simulink model "OEW_PMSM_DI_SVPWM_ZSC_Control"  (R2022b)
settings: Solver=FixedStepAuto  StartTime=0.0  StopTime=0.3  FixedStep=Ts  RelTol=1e-3
model workspace (MAT data in the model file):
  B = Simulink.Parameter
  B.Value = 0.002
  B.DataType = 'auto'
  B.Complexity = 'real'
  B.Dimensions = [1 1]
  J = Simulink.Parameter
  J.Value = 0.001
  J.DataType = 'auto'
  J.Complexity = 'real'
  J.Dimensions = [1 1]
  L0 = Simulink.Parameter
  L0.Value = 0.001
  L0.DataType = 'auto'
  L0.Complexity = 'real'
  L0.Dimensions = [1 1]
  Ld = Simulink.Parameter
  Ld.Value = 0.00176
  Ld.DataType = 'auto'
  Ld.Complexity = 'real'
  Ld.Dimensions = [1 1]
  Lq = Simulink.Parameter
  Lq.Value = 0.00176
  Lq.DataType = 'auto'
  Lq.Complexity = 'real'
  Lq.Dimensions = [1 1]
  Rs = Simulink.Parameter
  Rs.Value = 0.2
  Rs.DataType = 'auto'
  Rs.Complexity = 'real'
  Rs.Dimensions = [1 1]
  flux = Simulink.Parameter
  flux.Value = 0.1688
  flux.DataType = 'auto'
  flux.Complexity = 'real'
  flux.Dimensions = [1 1]
  flux_3 = Simulink.Parameter
  flux_3.Value = 0.006
  flux_3.DataType = 'auto'
  flux_3.Complexity = 'real'
  flux_3.Dimensions = [1 1]
  pn = Simulink.Parameter
  pn.Value = 4
  pn.DataType = 'auto'
  pn.Complexity = 'real'
  pn.Dimensions = [1 1]
undefined symbols (not defined in the file): DiscIntNeverNeededParam, Tpwm, Ts, Tsample, Tspeed, Udc
libraries: spsControlledCurrentSourceLib x3, spsVoltageMeasurementLib x3, slpidlib x3, spsUniversalBridgeLib x2, spsDCVoltageSourceLib x1, simulink x1, spsSecondOrderFilterLib x1, sps_lib x1
settings Model: DataDictionary=OEW_PMSM_DI_SVPWM_ZSC_Control.sldd  Creator=SSC  LastModifiedBy=SSC

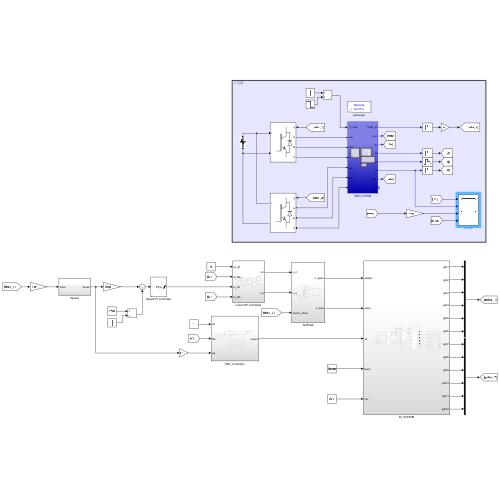
[thumbnail: Simulink's stored preview of the top-level diagram]
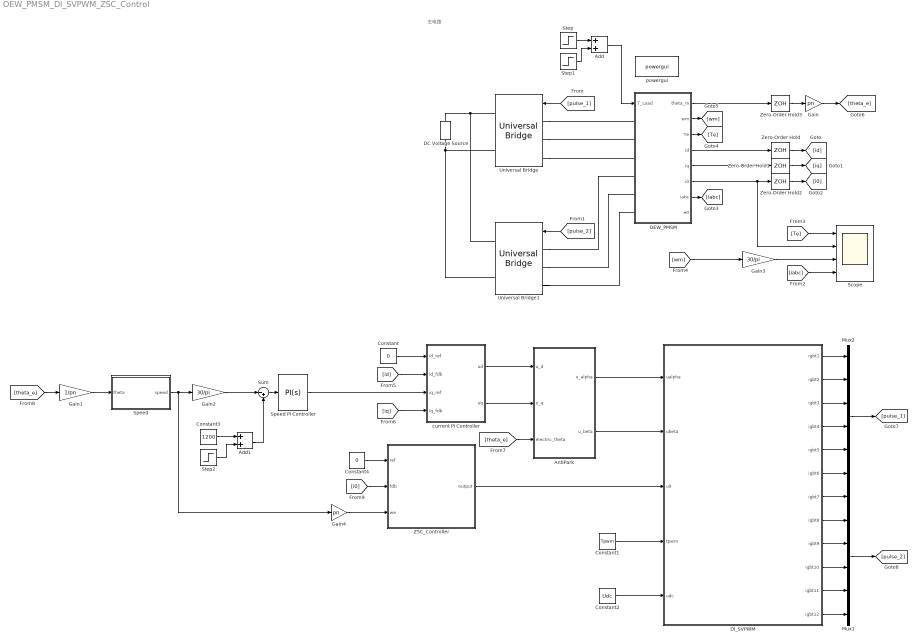
== system OEW_PMSM_DI_SVPWM_ZSC_Control ==
  note: 主电路
  Add : Sum
  Add1 : Sum
  AntiPark : Subsystem
  Constant : Constant  Value=0
  Constant1 : Constant  Value=Tpwm
  Constant2 : Constant  Value=Udc
  Constant3 : Constant  Value=1200
  Constant4 : Constant  Value=0
  DC Voltage Source : spsDCVoltageSourceLib/DC Voltage Source  Amplitude=Udc  Measurements=None
  DI_SVPWM : Subsystem
  Gain : Gain  Gain=pn
  Gain1 : Gain  Gain=1/pn
  Gain2 : Gain  Gain=30/pi
  Gain3 : Gain  Gain=30/pi
  Gain4 : Gain  Gain=pn
  Mux1 : Mux  Inputs=6
  Mux2 : Mux  Inputs=6
  OEW_PMSM : Subsystem
  Scope : Scope  NumInputPorts=4
  Speed : Subsystem
  Speed PI Controller : slpidlib/PID Controller  Controller=PI  Form=Parallel  TimeDomain=Continuous-time  UseExternalTs=off  SampleTime=1e-4  IntegratorMethod=Forward Euler  FilterMethod=Forward Euler  ControllerParametersSource=internal  P=0.1  I=40  UseKiTs=off  D=0  N=100  UseFilter=on  TunerSelectOption=Transfer Function Based (PID Tuner App)  InitialConditionSource=internal  InitialConditionForIntegrator=0  InitialConditionForFilter=0  DifferentiatorICPrevScaledInput=0  ExternalReset=none  TrackingMode=off  Kt=1  LimitOutput=on  SatLimitsSource=internal  UpperSaturationLimit=14  LowerSaturationLimit=-14  LinearizeAsGain=on  AntiWindupMode=clamping  Kb=1  LimitIntegrator=off  UpperIntegratorSaturationLimit=inf  LowerIntegratorSaturationLimit=-inf  POutMin=[]  POutMax=[]  IOutMin=[]  IOutMax=[]  DOutMin=[]  DOutMax=[]  NOutMin=[]  NOutMax=[]  SumOutMin=[]  SumOutMax=[]  SaturationOutMin=[]  SaturationOutMax=[]  PParamMin=[]  PParamMax=[]  IParamMin=[]  IParamMax=[]  DParamMin=[]  DParamMax=[]  NParamMin=[]  NParamMax=[]  KbParamMin=[]  KbParamMax=[]  KtParamMin=[]  KtParamMax=[]  KbOutMin=[]  KbOutMax=[]  KtOutMin=[]  KtOutMax=[]  IntegratorOutMin=[]  IntegratorOutMax=[]  FilterOutMin=[]  FilterOutMax=[]  SumI1OutMin=[]  SumI1OutMax=[]  SumI2OutMin=[]  SumI2OutMax=[]  SumI3OutMin=[]  SumI3OutMax=[]  SumI4OutMin=[]  SumI4OutMax=[]  SumDOutMin=[]  SumDOutMax=[]  DifferentiatorOutMin=[]  DifferentiatorOutMax=[]  FilterDiffOutCoefMin=[]  FilterDiffOutCoefMax=[]  ReciprocalOutMin=[]  ReciprocalOutMax=[]  SumDenOutMin=[]  SumDenOutMax=[]  SumNumOutMin=[]  SumNumOutMax=[]  DivideOutMin=[]  DivideOutMax=[]  UdiffTsProdOutMin=[]  UdiffTsProdOutMax=[]  NTsProdOutMin=[]  NTsProdOutMax=[]  UintegralTsProdOutMin=[]  UintegralTsProdOutMax=[]  UngainTsProdOutMin=[]  UngainTsProdOutMax=[]  ClampingZeroOutDataTypeStr=Inherit: Inherit via back propagation  ClampingZeroOutMin=[]  ClampingZeroOutMax=[]  FilterDenConstantOutDataTypeStr=Inherit: Inherit via back propagation  FilterDenConstantOutMin=[]  FilterDenConstantOutMax=[]  PCopyOutDataTypeStr=Inherit: Inherit via back propagation  PCopyOutMin=[]  PCopyOutMax=[]  NCopyOutDataTypeStr=Inherit: Inherit via back propagation  NCopyOutMin=[]  NCopyOutMax=[]  IntegratorContinuousStateAttributes=''  IntegratorStateMustResolveToSignalObject=off  IntegratorRTWStateStorageClass=Auto  FilterContinuousStateAttributes=''  FilterStateMustResolveToSignalObject=off  FilterRTWStateStorageClass=Auto  ParallelPVariant=InternalParameters  IdealPVariant=Disabled  IVariant=InternalParameters  DVariant=Disabled  IntegratorVariant=Continuous  SatVariant=Enabled  AWVariant=ContClampingParallel  PCopyVariant=Disabled  TRVariant=Disabled  FdbkBlocksVariant=Forward  IdealPFdbkVariant=Disabled  SatFdbkVariant=Disabled  DerivativeFilterVariant=Disabled  NVariant=Disabled  NCopyVariant=Disabled_SignalSpec  FilterICVariant=Disabled  IntegratorICVariant=InternalICs  ExternalResetVariant=Disabled  TRSumVariant=Passthrough  SumFdbkVariant=Disabled  SumVariant=Sum_PI  TsampFilterVariant=InternalTs  TsampNgainVariant=Passthrough  TsampIntegralVariant=Passthrough  ExternalSaturationOutDataTypeStr=Inherit: Same as second input
  Step : Step  Time=0.05  After=12  SampleTime=0
  Step1 : Step  Time=0.12  After=-6  SampleTime=0
  Step2 : Step  Time=0.15  After=-600  SampleTime=0
  Sum : Sum  Inputs=|-+
  Universal Bridge : spsUniversalBridgeLib/Universal Bridge  Arms=3  SnubberResistance=1e5  SnubberCapacitance=inf  Device=IGBT / Diodes  Ron=1e-3  Lon=0  ForwardVoltages="[  0  0  ]"  ForwardVoltage=0  GTOparameters=[ 10e-6 , 20e-6 ]  IGBTparameters=[ 1e-6 , 2e-6 ]  Measurements=None  Measurements_2=None  converterType=Rectifier
  Universal Bridge1 : spsUniversalBridgeLib/Universal Bridge  Arms=3  SnubberResistance=1e5  SnubberCapacitance=inf  Device=IGBT / Diodes  Ron=1e-3  Lon=0  ForwardVoltages="[  0  0  ]"  ForwardVoltage=0  GTOparameters=[ 10e-6 , 20e-6 ]  IGBTparameters=[ 1e-6 , 2e-6 ]  Measurements=None  Measurements_2=None  converterType=Rectifier
  ZSC_Controller : Subsystem
  Zero-Order Hold{,1..3} (4 alike) : ZeroOrderHold  SampleTime=Tsample
  current PI Controller : Subsystem
  powergui : sps_lib/powergui  Priority=1  SimulationMode=Discrete  SampleTime=Ts  frequency=60  Iterations=50  frequencyindice=0  Pbase=100e6  ErrMax=1e-4  UnitsV=kV  UnitsW=MW  buscounter=0  FunctionMessages=off  echomessages=off  EnableUseOfTLC=off  CurrentSourceSwitches=off  DisableSnubberDevices=off  DisableRonSwitches=off  DisableVfSwitches=off  DisplayEquations=off  AutomaticDiscreteSolvers=off  SolverType=Tustin/Backward Euler (TBE)  Interpol=off  ExternalGateDelay=off  methode=off  Ts=100  x0status=blocks  SPID=on  SwTol=0  HookPort=off  NonlinearTolerance=1e-4  nMaxIteration=100  ContinueOnMaxIteration=off  RestoreLinks=warning  ResistiveCurrentMeasurement=off  Frange=[0:2:500]  Ylog=off  Xlog=on  ShowGrid=off  save=off  variable=ZData  structure=0  ZoomFFT=off  StartTime=0.0  cycles=1  DisplayStyle=1  fundamental=60  FreqAxis=off  MaxFrequency=1000  frequencyindicesteady=1  RmsSteady=1  display=off
  wires:
  [pulse_1] -> Universal Bridge/1
  [pulse_2] -> Universal Bridge1/1
  OEW_PMSM/4(id) -> Zero-Order Hold/1
  OEW_PMSM/5(iq) -> Zero-Order Hold1/1
  OEW_PMSM/6(i0) -> Scope/2, Zero-Order Hold2/1
  Zero-Order Hold/1 -> [id]
  Zero-Order Hold1/1 -> [iq]
  Zero-Order Hold2/1 -> [i0]
  OEW_PMSM/7(iabc) -> [iabc]
  [iabc] -> Scope/4
  OEW_PMSM/3(Te) -> [Te]
  [Te] -> Scope/1
  OEW_PMSM/2(wm) -> [wm]
  [wm] -> Gain3/1
  OEW_PMSM/1(theta_m) -> Zero-Order Hold3/1
  Zero-Order Hold3/1 -> Gain/1
  Gain/1 -> [theta_e]
  Step1/1 -> Add/2
  Step/1 -> Add/1
  Add/1 -> OEW_PMSM/1(T_Load)
  Constant/1 -> current PI Controller/1(id_ref)
  [id] -> current PI Controller/2(id_fdb)
  [iq] -> current PI Controller/4(iq_fdb)
  current PI Controller/1(ud) -> AntiPark/1(u_d)
  current PI Controller/2(uq) -> AntiPark/2(u_q)
  [theta_e] -> AntiPark/3(electric_theta)
  AntiPark/1(u_alpha) -> DI_SVPWM/1(ualpha)
  AntiPark/2(u_beta) -> DI_SVPWM/2(ubeta)
  Gain1/1 -> Speed/1(theta)
  [theta_e] -> Gain1/1
  Speed/1(speed) -> Gain4/1, Gain2/1
  Gain2/1 -> Sum/1
  Constant3/1 -> Add1/1
  Sum/1 -> Speed PI Controller/1
  Add1/1 -> Sum/2
  Step2/1 -> Add1/2
  Speed PI Controller/1 -> current PI Controller/3(iq_ref)
  Gain3/1 -> Scope/3
  Constant1/1 -> DI_SVPWM/4(tpwm)
  Constant2/1 -> DI_SVPWM/5(udc)
  DI_SVPWM/12(igbt12) -> Mux1/6
  DI_SVPWM/11(igbt11) -> Mux1/5
  DI_SVPWM/10(igbt10) -> Mux1/4
  DI_SVPWM/9(igbt9) -> Mux1/3
  DI_SVPWM/8(igbt8) -> Mux1/2
  DI_SVPWM/7(igbt7) -> Mux1/1
  DI_SVPWM/6(igbt6) -> Mux2/6
  DI_SVPWM/5(igbt5) -> Mux2/5
  DI_SVPWM/4(igbt4) -> Mux2/4
  DI_SVPWM/3(igbt3) -> Mux2/3
  DI_SVPWM/2(igbt2) -> Mux2/2
  DI_SVPWM/1(igbt1) -> Mux2/1
  Mux2/1 -> [pulse_1]
  Mux1/1 -> [pulse_2]
  ZSC_Controller/1(output) -> DI_SVPWM/3(u0)
  Constant4/1 -> ZSC_Controller/1(ref)
  [i0] -> ZSC_Controller/2(fdb)
  Gain4/1 -> ZSC_Controller/3(we)
  connections:
  Universal Bridge/LConn1 -- OEW_PMSM/LConn1
  Universal Bridge/LConn2 -- OEW_PMSM/LConn2
  Universal Bridge/LConn3 -- OEW_PMSM/LConn3
  Universal Bridge1/LConn1 -- OEW_PMSM/LConn4
  Universal Bridge1/LConn2 -- OEW_PMSM/LConn5
  Universal Bridge1/LConn3 -- OEW_PMSM/LConn6
  DC Voltage Source/LConn1 -- Universal Bridge/RConn2 -- Universal Bridge1/RConn2
  Universal Bridge1/RConn1 -- Universal Bridge/RConn1 -- DC Voltage Source/RConn1

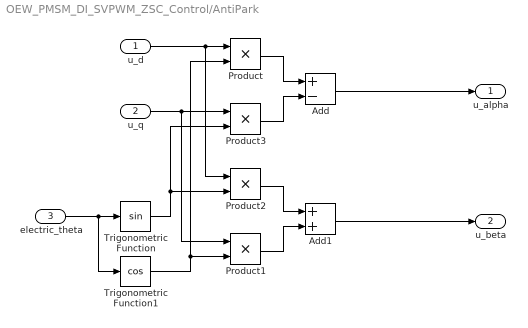
== system OEW_PMSM_DI_SVPWM_ZSC_Control/AntiPark ==
  u_d : Inport
  u_q : Inport  Port=2
  electric_theta : Inport  Port=3
  Add : Sum  Inputs=+-
  Add1 : Sum
  Product{,1..3} (4 alike) : Product
  Trigonometric Function : Trigonometry
  Trigonometric Function1 : Trigonometry  Operator=cos
  u_alpha : Outport
  u_beta : Outport  Port=2
  wires:
  electric_theta/1 -> Trigonometric Function1/1, Trigonometric Function/1
  u_d/1 -> Product2/1, Product/1
  Trigonometric Function1/1 -> Product/2, Product1/2
  u_q/1 -> Product1/1, Product3/1
  Trigonometric Function/1 -> Product2/2, Product3/2
  Product/1 -> Add/1
  Product3/1 -> Add/2
  Add/1 -> u_alpha/1
  Product2/1 -> Add1/1
  Product1/1 -> Add1/2
  Add1/1 -> u_beta/1

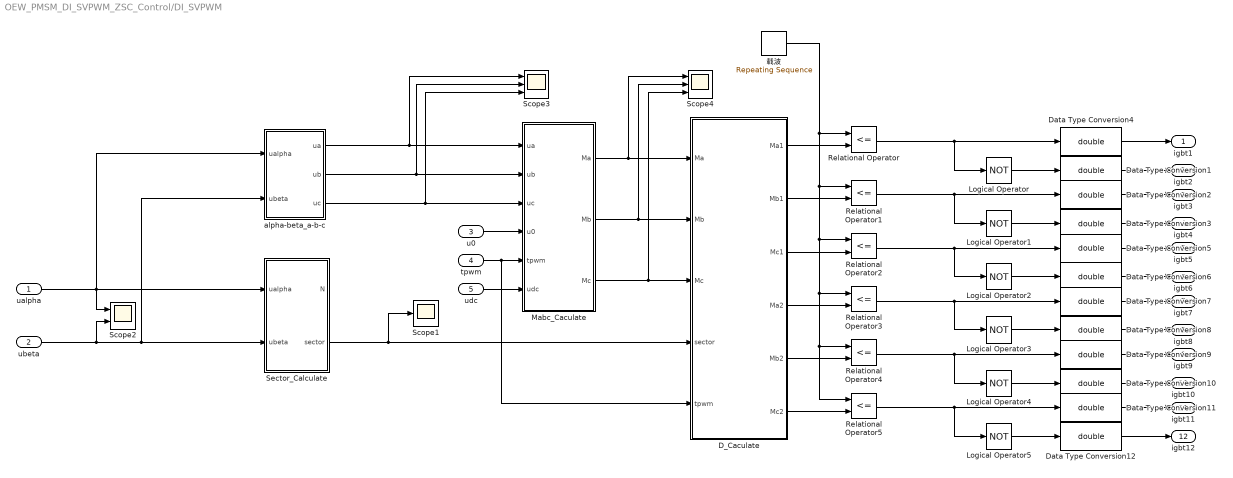
== system OEW_PMSM_DI_SVPWM_ZSC_Control/DI_SVPWM ==
  ualpha : Inport
  ubeta : Inport  Port=2
  u0 : Inport  Port=3
  tpwm : Inport  Port=4
  udc : Inport  Port=5
  D_Caculate : MATLAB Function  TreatAsAtomicUnit=on
  Data Type Conversion{1..12} (12 alike) : DataTypeConversion  OutDataTypeStr=double  SaturateOnIntegerOverflow=off  RndMeth=Floor
  Logical Operator{,1..5} (6 alike) : Logic  Operator=NOT  AllPortsSameDT=off  OutDataTypeStr=boolean
  Mabc_Caculate : MATLAB Function  TreatAsAtomicUnit=on
  Relational Operator{,1..5} (6 alike) : RelationalOperator  Operator=<=  OutDataTypeStr=boolean  RndMeth=Simplest  InputSameDT=off
  Scope1 : Scope
  Scope2 : Scope  NumInputPorts=2
  Scope3 : Scope  NumInputPorts=3
  Scope4 : Scope  NumInputPorts=3
  Sector_Calculate : Subsystem
  alpha-beta_a-b-c : Subsystem
  载波 : simulink/Sources/Repeating Sequence  rep_seq_t=[0 0.5*(1e-4) 1e-4]  rep_seq_y=[0 1e-4 0]
  igbt1 : Outport
  igbt2 : Outport  Port=2
  igbt3 : Outport  Port=3
  igbt4 : Outport  Port=4
  igbt5 : Outport  Port=5
  igbt6 : Outport  Port=6
  igbt7 : Outport  Port=7
  igbt8 : Outport  Port=8
  igbt9 : Outport  Port=9
  igbt10 : Outport  Port=10
  igbt11 : Outport  Port=11
  igbt12 : Outport  Port=12
  wires:
  ubeta/1 -> Scope2/2, alpha-beta_a-b-c/2(ubeta), Sector_Calculate/2(ubeta)
  ualpha/1 -> Scope2/1, Sector_Calculate/1(ualpha), alpha-beta_a-b-c/1(ualpha)
  alpha-beta_a-b-c/1(ua) -> Scope3/1, Mabc_Caculate/1(ua)
  alpha-beta_a-b-c/2(ub) -> Scope3/2, Mabc_Caculate/2(ub)
  alpha-beta_a-b-c/3(uc) -> Scope3/3, Mabc_Caculate/3(uc)
  tpwm/1 -> D_Caculate/5(tpwm), Mabc_Caculate/5(tpwm)
  udc/1 -> Mabc_Caculate/6(udc)
  Mabc_Caculate/1(Ma) -> Scope4/1, D_Caculate/1(Ma)
  Mabc_Caculate/2(Mb) -> Scope4/2, D_Caculate/2(Mb)
  Mabc_Caculate/3(Mc) -> Scope4/3, D_Caculate/3(Mc)
  Sector_Calculate/2(sector) -> D_Caculate/4(sector), Scope1/1
  D_Caculate/1(Ma1) -> Relational Operator/2
  D_Caculate/3(Mc1) -> Relational Operator2/2
  D_Caculate/2(Mb1) -> Relational Operator1/2
  D_Caculate/4(Ma2) -> Relational Operator3/2
  D_Caculate/5(Mb2) -> Relational Operator4/2
  D_Caculate/6(Mc2) -> Relational Operator5/2
  载波/1 -> Relational Operator1/1, Relational Operator2/1, Relational Operator3/1, Relational Operator5/1, Relational Operator4/1, Relational Operator/1
  Relational Operator/1 -> Logical Operator/1, Data Type Conversion4/1
  Logical Operator/1 -> Data Type Conversion1/1
  Relational Operator1/1 -> Logical Operator1/1, Data Type Conversion2/1
  Logical Operator1/1 -> Data Type Conversion3/1
  Relational Operator2/1 -> Logical Operator2/1, Data Type Conversion5/1
  Logical Operator2/1 -> Data Type Conversion6/1
  Relational Operator3/1 -> Logical Operator3/1, Data Type Conversion7/1
  Logical Operator3/1 -> Data Type Conversion8/1
  Relational Operator4/1 -> Logical Operator4/1, Data Type Conversion9/1
  Logical Operator4/1 -> Data Type Conversion10/1
  Relational Operator5/1 -> Logical Operator5/1, Data Type Conversion11/1
  Logical Operator5/1 -> Data Type Conversion12/1
  u0/1 -> Mabc_Caculate/4(u0)
  Data Type Conversion4/1 -> igbt1/1
  Data Type Conversion1/1 -> igbt2/1
  Data Type Conversion2/1 -> igbt3/1
  Data Type Conversion3/1 -> igbt4/1
  Data Type Conversion5/1 -> igbt5/1
  Data Type Conversion6/1 -> igbt6/1
  Data Type Conversion7/1 -> igbt7/1
  Data Type Conversion8/1 -> igbt8/1
  Data Type Conversion9/1 -> igbt9/1
  Data Type Conversion10/1 -> igbt10/1
  Data Type Conversion11/1 -> igbt11/1
  Data Type Conversion12/1 -> igbt12/1

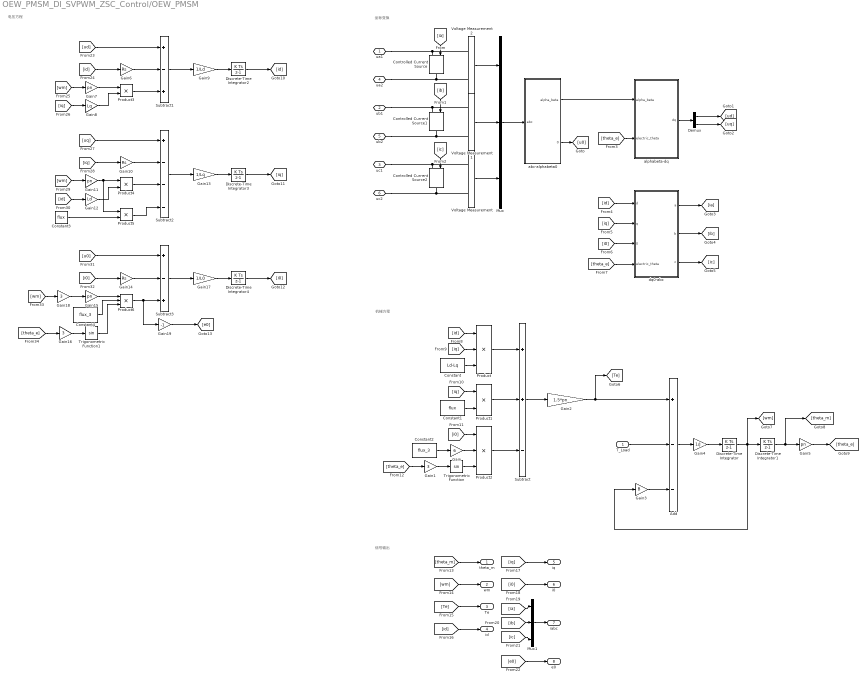
== system OEW_PMSM_DI_SVPWM_ZSC_Control/OEW_PMSM ==
  note: 电压方程
  note: 信号输出
  note: 机械方程
  note: 坐标变换
  T_Load : Inport
  Add : Sum  Inputs=+--
  Constant : Constant  Value=Ld-Lq
  Constant1 : Constant  Value=flux
  Constant2 : Constant  Value=flux_3
  Constant3 : Constant  Value=flux
  Constant4 : Constant  Value=flux_3
  Controlled Current Source : spsControlledCurrentSourceLib/Controlled Current Source  Initialize=on  Source_Type=AC  Amplitude=0  Phase=0  Frequency=0  Measurements=None
  Controlled Current Source1 : spsControlledCurrentSourceLib/Controlled Current Source  Initialize=on  Source_Type=AC  Amplitude=0  Phase=0  Frequency=0  Measurements=None
  Controlled Current Source2 : spsControlledCurrentSourceLib/Controlled Current Source  Initialize=on  Source_Type=AC  Amplitude=0  Phase=0  Frequency=0  Measurements=None
  Demux : Demux  Outputs=2
  Discrete-Time Integrator{,1..4} (5 alike) : DiscreteIntegrator  SampleTime=Ts  ICPrevOutput=DiscIntNeverNeededParam  ICPrevScaledInput=DiscIntNeverNeededParam
  Gain : Gain  Gain=6
  Gain1 : Gain  Gain=3
  Gain10 : Gain  Gain=Rs
  Gain{5,7,11,15} (4 alike) : Gain  Gain=pn
  Gain12 : Gain  Gain=Ld
  Gain13 : Gain  Gain=1/Lq
  Gain14 : Gain  Gain=Rs
  Gain16 : Gain  Gain=3
  Gain17 : Gain  Gain=1/L0
  Gain18 : Gain  Gain=3
  Gain19 : Gain  Gain=-1
  Gain2 : Gain  Gain=1.5*pn
  Gain3 : Gain  Gain=B
  Gain4 : Gain  Gain=1/J
  Gain6 : Gain  Gain=Rs
  Gain8 : Gain  Gain=Lq
  Gain9 : Gain  Gain=1/Ld
  Mux : Mux  Inputs=3
  Mux1 : Mux  Inputs=3
  Product : Product  Inputs=3
  Product{1,3..5} (4 alike) : Product
  Product2 : Product  Inputs=3
  Product6 : Product  Inputs=3
  Subtract : Sum  Inputs=++-
  Subtract1 : Sum  Inputs=+-+
  Subtract2 : Sum  Inputs=+---
  Subtract3 : Sum  Inputs=+-+
  Trigonometric Function : Trigonometry
  Trigonometric Function1 : Trigonometry
  Voltage Measurement : spsVoltageMeasurementLib/Voltage Measurement  PhasorSimulation=off  OutputType=Complex  PSBequivalent=0
  Voltage Measurement1 : spsVoltageMeasurementLib/Voltage Measurement  PhasorSimulation=off  OutputType=Complex  PSBequivalent=0
  Voltage Measurement2 : spsVoltageMeasurementLib/Voltage Measurement  PhasorSimulation=off  OutputType=Complex  PSBequivalent=0
  abc-alphabeta0 : Subsystem
  alphabeta-dq : Subsystem
  dq0-abc : Subsystem
  ua1 : PMIOPort  Side=Left
  ub1 : PMIOPort  Port=2  Side=Left
  uc1 : PMIOPort  Port=3  Side=Left
  ua2 : PMIOPort  Port=4  Side=Left
  ub2 : PMIOPort  Port=5  Side=Left
  uc2 : PMIOPort  Port=6  Side=Left
  theta_m : Outport
  wm : Outport  Port=2
  Te : Outport  Port=3
  id : Outport  Port=4
  iq : Outport  Port=5
  i0 : Outport  Port=6
  iabc : Outport  Port=7
  e0 : Outport  Port=8
  wires:
  [id] -> Gain12/1
  [id] -> Product/1
  [iq] -> Product/2
  [i0] -> Gain14/1
  alphabeta-dq/1(dq) -> Demux/1
  Gain12/1 -> Product4/2
  Gain19/1 -> [e0]
  [ia] -> Mux1/1
  [iq] -> Gain8/1
  abc-alphabeta0/1(alpha_beta) -> alphabeta-dq/1(alpha_beta)
  Product3/1 -> Subtract1/3
  Subtract2/1 -> Gain13/1
  Gain6/1 -> Subtract1/2
  Product1/1 -> Subtract/2
  Demux/1 -> [ud]
  [theta_e] -> alphabeta-dq/2(electric_theta)
  Gain13/1 -> Discrete-Time Integrator3/1
  Constant1/1 -> Product1/2
  Subtract1/1 -> Gain9/1
  Voltage Measurement1/1 -> Mux/2
  Gain11/1 -> Product5/1, Product4/1
  [ic] -> Controlled Current Source2/1
  dq0-abc/1(a) -> [ia]
  Mux/1 -> abc-alphabeta0/1(abc)
  [iq] -> Gain10/1
  Gain4/1 -> Discrete-Time Integrator/1
  [ib] -> Controlled Current Source1/1
  Demux/2 -> [uq]
  [theta_e] -> Gain16/1
  [ic] -> Mux1/3
  Voltage Measurement/1 -> Mux/3
  Gain3/1 -> Add/3
  Product4/1 -> Subtract2/3
  [iq] -> iq/1
  Gain16/1 -> Trigonometric Function1/1
  [ia] -> Controlled Current Source/1
  Gain1/1 -> Trigonometric Function/1
  abc-alphabeta0/2(0) -> [u0]
  dq0-abc/3(c) -> [ic]
  dq0-abc/2(b) -> [ib]
  T_Load/1 -> Add/2
  [ud] -> Subtract1/1
  Discrete-Time Integrator3/1 -> [iq]
  Voltage Measurement2/1 -> Mux/1
  Constant3/1 -> Product5/2
  Subtract3/1 -> Gain17/1
  Constant/1 -> Product/3
  [iq] -> dq0-abc/2(q)
  [uq] -> Subtract2/1
  Add/1 -> Gain4/1
  [theta_e] -> dq0-abc/4(electric_theta)
  [i0] -> dq0-abc/3(0)
  Product6/1 -> Subtract3/3, Gain19/1
  [id] -> dq0-abc/1(d)
  [wm] -> wm/1
  Discrete-Time Integrator/1 -> Discrete-Time Integrator1/1, Gain3/1, [wm]
  [iq] -> Product1/1
  [wm] -> Gain7/1
  Product/1 -> Subtract/1
  Gain10/1 -> Subtract2/2
  [wm] -> Gain11/1
  Product5/1 -> Subtract2/4
  Constant4/1 -> Product6/2
  Mux1/1 -> iabc/1
  Gain18/1 -> Gain15/1
  Gain5/1 -> [theta_e]
  Trigonometric Function1/1 -> Product6/3
  Gain9/1 -> Discrete-Time Integrator2/1
  Gain7/1 -> Product3/1
  Trigonometric Function/1 -> Product2/3
  Discrete-Time Integrator1/1 -> Gain5/1, [theta_m]
  [ib] -> Mux1/2
  [theta_e] -> Gain1/1
  Gain8/1 -> Product3/2
  [Te] -> Te/1
  Product2/1 -> Subtract/3
  [i0] -> Product2/1
  Discrete-Time Integrator2/1 -> [id]
  [id] -> Gain6/1
  Gain/1 -> Product2/2
  Gain2/1 -> Add/1, [Te]
  Constant2/1 -> Gain/1
  Subtract/1 -> Gain2/1
  [theta_m] -> theta_m/1
  Discrete-Time Integrator4/1 -> [i0]
  Gain17/1 -> Discrete-Time Integrator4/1
  Gain15/1 -> Product6/1
  [u0] -> Subtract3/1
  Gain14/1 -> Subtract3/2
  [wm] -> Gain18/1
  [i0] -> i0/1
  [id] -> id/1
  [e0] -> e0/1
  connections:
  Voltage Measurement2/LConn2 -- ua2/RConn1 -- Controlled Current Source/RConn1
  Voltage Measurement1/LConn2 -- ub2/RConn1 -- Controlled Current Source1/RConn1
  Voltage Measurement2/LConn1 -- ua1/RConn1 -- Controlled Current Source/LConn1
  Voltage Measurement/LConn2 -- uc2/RConn1 -- Controlled Current Source2/RConn1
  Voltage Measurement1/LConn1 -- ub1/RConn1 -- Controlled Current Source1/LConn1
  Voltage Measurement/LConn1 -- uc1/RConn1 -- Controlled Current Source2/LConn1

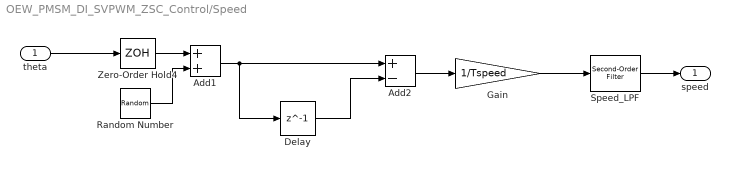
== system OEW_PMSM_DI_SVPWM_ZSC_Control/Speed ==
  theta : Inport
  Add1 : Sum
  Add2 : Sum  Inputs=+-
  Delay : Delay  DelayLength=1  InitialCondition=0  SampleTime=Tspeed
  Gain : Gain  Gain=1/Tspeed
  Random Number : RandomNumber  Mean=2.5e-10  Variance=2.5e-10  SampleTime=Tspeed
  Speed_LPF : spsSecondOrderFilterLib/Second-Order Filter  FilterType=Lowpass  Fo=500  Zeta=0.707  Ts=Tspeed  Initialize=off  Vac_Init="[0,  0,  60]"  Vdc_Init=0  PlotResponse=off  FreqRange=[0, 500, 1]
      settings: LibrarySourceBlock=|
      | sps_lib/Control/Filters/Second-Order
      | Filter
  Zero-Order Hold4 : ZeroOrderHold  SampleTime=Tspeed
  speed : Outport
  wires:
  Zero-Order Hold4/1 -> Add1/1
  Random Number/1 -> Add1/2
  theta/1 -> Zero-Order Hold4/1
  Speed_LPF/1 -> speed/1
  Add2/1 -> Gain/1
  Gain/1 -> Speed_LPF/1
  Add1/1 -> Delay/1, Add2/1
  Delay/1 -> Add2/2

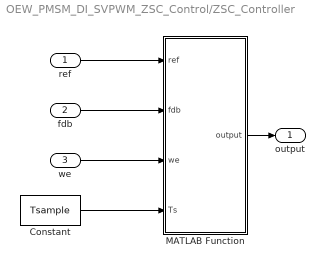
== system OEW_PMSM_DI_SVPWM_ZSC_Control/ZSC_Controller ==
  ref : Inport
  fdb : Inport  Port=2
  we : Inport  Port=3
  Constant : Constant  Value=Tsample
  MATLAB Function : MATLAB Function  TreatAsAtomicUnit=on
  output : Outport
  wires:
  MATLAB Function/1(output) -> output/1
  ref/1 -> MATLAB Function/1(ref)
  fdb/1 -> MATLAB Function/2(fdb)
  we/1 -> MATLAB Function/3(we)
  Constant/1 -> MATLAB Function/4(Ts)

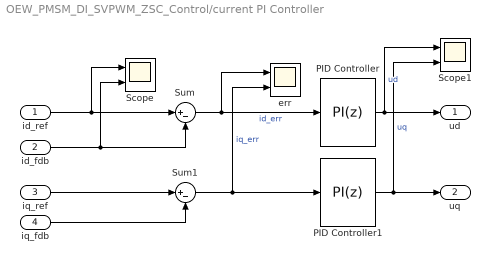
== system OEW_PMSM_DI_SVPWM_ZSC_Control/current PI Controller ==
  id_ref : Inport
  id_fdb : Inport  Port=2
  iq_ref : Inport  Port=3
  iq_fdb : Inport  Port=4
  PID Controller : slpidlib/PID Controller  Controller=PI  Form=Parallel  TimeDomain=Discrete-time  UseExternalTs=off  SampleTime=Tsample  IntegratorMethod=Forward Euler  FilterMethod=Forward Euler  ControllerParametersSource=internal  P=5.5292  I=628.32  UseKiTs=off  D=0  N=100  UseFilter=on  TunerSelectOption=Transfer Function Based (PID Tuner App)  InitialConditionSource=internal  InitialConditionForIntegrator=0  InitialConditionForFilter=0  DifferentiatorICPrevScaledInput=0  ExternalReset=none  TrackingMode=off  Kt=1  LimitOutput=on  SatLimitsSource=internal  UpperSaturationLimit=Udc  LowerSaturationLimit=-Udc  LinearizeAsGain=on  AntiWindupMode=clamping  Kb=1  LimitIntegrator=off  UpperIntegratorSaturationLimit=inf  LowerIntegratorSaturationLimit=-inf  POutMin=[]  POutMax=[]  IOutMin=[]  IOutMax=[]  DOutMin=[]  DOutMax=[]  NOutMin=[]  NOutMax=[]  SumOutMin=[]  SumOutMax=[]  SaturationOutMin=[]  SaturationOutMax=[]  PParamMin=[]  PParamMax=[]  IParamMin=[]  IParamMax=[]  DParamMin=[]  DParamMax=[]  NParamMin=[]  NParamMax=[]  KbParamMin=[]  KbParamMax=[]  KtParamMin=[]  KtParamMax=[]  KbOutMin=[]  KbOutMax=[]  KtOutMin=[]  KtOutMax=[]  IntegratorOutMin=[]  IntegratorOutMax=[]  FilterOutMin=[]  FilterOutMax=[]  SumI1OutMin=[]  SumI1OutMax=[]  SumI2OutMin=[]  SumI2OutMax=[]  SumI3OutMin=[]  SumI3OutMax=[]  SumI4OutMin=[]  SumI4OutMax=[]  SumDOutMin=[]  SumDOutMax=[]  DifferentiatorOutMin=[]  DifferentiatorOutMax=[]  FilterDiffOutCoefMin=[]  FilterDiffOutCoefMax=[]  ReciprocalOutMin=[]  ReciprocalOutMax=[]  SumDenOutMin=[]  SumDenOutMax=[]  SumNumOutMin=[]  SumNumOutMax=[]  DivideOutMin=[]  DivideOutMax=[]  UdiffTsProdOutMin=[]  UdiffTsProdOutMax=[]  NTsProdOutMin=[]  NTsProdOutMax=[]  UintegralTsProdOutMin=[]  UintegralTsProdOutMax=[]  UngainTsProdOutMin=[]  UngainTsProdOutMax=[]  ClampingZeroOutDataTypeStr=Inherit: Inherit via back propagation  ClampingZeroOutMin=[]  ClampingZeroOutMax=[]  FilterDenConstantOutDataTypeStr=Inherit: Inherit via back propagation  FilterDenConstantOutMin=[]  FilterDenConstantOutMax=[]  PCopyOutDataTypeStr=Inherit: Inherit via back propagation  PCopyOutMin=[]  PCopyOutMax=[]  NCopyOutDataTypeStr=Inherit: Inherit via back propagation  NCopyOutMin=[]  NCopyOutMax=[]  IntegratorContinuousStateAttributes=''  IntegratorStateMustResolveToSignalObject=off  IntegratorRTWStateStorageClass=Auto  FilterContinuousStateAttributes=''  FilterStateMustResolveToSignalObject=off  FilterRTWStateStorageClass=Auto  ParallelPVariant=InternalParameters  IdealPVariant=Disabled  IVariant=InternalParameters  DVariant=Disabled  IntegratorVariant=Discrete  SatVariant=Enabled  AWVariant=DiscClampingParallel  PCopyVariant=Disabled  TRVariant=Disabled  FdbkBlocksVariant=Forward  IdealPFdbkVariant=Disabled  SatFdbkVariant=Disabled  DerivativeFilterVariant=Disabled  NVariant=Disabled  NCopyVariant=Disabled_SignalSpec  FilterICVariant=Disabled  IntegratorICVariant=InternalICs  ExternalResetVariant=Disabled  TRSumVariant=Passthrough  SumFdbkVariant=Disabled  SumVariant=Sum_PI  TsampFilterVariant=InternalTs  TsampNgainVariant=Passthrough  TsampIntegralVariant=Passthrough  ExternalSaturationOutDataTypeStr=Inherit: Same as second input
  PID Controller1 : slpidlib/PID Controller  Controller=PI  Form=Parallel  TimeDomain=Discrete-time  UseExternalTs=off  SampleTime=Tsample  IntegratorMethod=Forward Euler  FilterMethod=Forward Euler  ControllerParametersSource=internal  P=5.5292  I=628.32  UseKiTs=off  D=0  N=100  UseFilter=on  TunerSelectOption=Transfer Function Based (PID Tuner App)  InitialConditionSource=internal  InitialConditionForIntegrator=0  InitialConditionForFilter=0  DifferentiatorICPrevScaledInput=0  ExternalReset=none  TrackingMode=off  Kt=1  LimitOutput=on  SatLimitsSource=internal  UpperSaturationLimit=Udc  LowerSaturationLimit=-Udc  LinearizeAsGain=on  AntiWindupMode=clamping  Kb=1  LimitIntegrator=off  UpperIntegratorSaturationLimit=inf  LowerIntegratorSaturationLimit=-inf  POutMin=[]  POutMax=[]  IOutMin=[]  IOutMax=[]  DOutMin=[]  DOutMax=[]  NOutMin=[]  NOutMax=[]  SumOutMin=[]  SumOutMax=[]  SaturationOutMin=[]  SaturationOutMax=[]  PParamMin=[]  PParamMax=[]  IParamMin=[]  IParamMax=[]  DParamMin=[]  DParamMax=[]  NParamMin=[]  NParamMax=[]  KbParamMin=[]  KbParamMax=[]  KtParamMin=[]  KtParamMax=[]  KbOutMin=[]  KbOutMax=[]  KtOutMin=[]  KtOutMax=[]  IntegratorOutMin=[]  IntegratorOutMax=[]  FilterOutMin=[]  FilterOutMax=[]  SumI1OutMin=[]  SumI1OutMax=[]  SumI2OutMin=[]  SumI2OutMax=[]  SumI3OutMin=[]  SumI3OutMax=[]  SumI4OutMin=[]  SumI4OutMax=[]  SumDOutMin=[]  SumDOutMax=[]  DifferentiatorOutMin=[]  DifferentiatorOutMax=[]  FilterDiffOutCoefMin=[]  FilterDiffOutCoefMax=[]  ReciprocalOutMin=[]  ReciprocalOutMax=[]  SumDenOutMin=[]  SumDenOutMax=[]  SumNumOutMin=[]  SumNumOutMax=[]  DivideOutMin=[]  DivideOutMax=[]  UdiffTsProdOutMin=[]  UdiffTsProdOutMax=[]  NTsProdOutMin=[]  NTsProdOutMax=[]  UintegralTsProdOutMin=[]  UintegralTsProdOutMax=[]  UngainTsProdOutMin=[]  UngainTsProdOutMax=[]  ClampingZeroOutDataTypeStr=Inherit: Inherit via back propagation  ClampingZeroOutMin=[]  ClampingZeroOutMax=[]  FilterDenConstantOutDataTypeStr=Inherit: Inherit via back propagation  FilterDenConstantOutMin=[]  FilterDenConstantOutMax=[]  PCopyOutDataTypeStr=Inherit: Inherit via back propagation  PCopyOutMin=[]  PCopyOutMax=[]  NCopyOutDataTypeStr=Inherit: Inherit via back propagation  NCopyOutMin=[]  NCopyOutMax=[]  IntegratorContinuousStateAttributes=''  IntegratorStateMustResolveToSignalObject=off  IntegratorRTWStateStorageClass=Auto  FilterContinuousStateAttributes=''  FilterStateMustResolveToSignalObject=off  FilterRTWStateStorageClass=Auto  ParallelPVariant=InternalParameters  IdealPVariant=Disabled  IVariant=InternalParameters  DVariant=Disabled  IntegratorVariant=Discrete  SatVariant=Enabled  AWVariant=DiscClampingParallel  PCopyVariant=Disabled  TRVariant=Disabled  FdbkBlocksVariant=Forward  IdealPFdbkVariant=Disabled  SatFdbkVariant=Disabled  DerivativeFilterVariant=Disabled  NVariant=Disabled  NCopyVariant=Disabled_SignalSpec  FilterICVariant=Disabled  IntegratorICVariant=InternalICs  ExternalResetVariant=Disabled  TRSumVariant=Passthrough  SumFdbkVariant=Disabled  SumVariant=Sum_PI  TsampFilterVariant=InternalTs  TsampNgainVariant=Passthrough  TsampIntegralVariant=Passthrough  ExternalSaturationOutDataTypeStr=Inherit: Same as second input
  Scope : Scope  NumInputPorts=2
  Scope1 : Scope  NumInputPorts=2
  Sum : Sum  Inputs=|+-
  Sum1 : Sum  Inputs=|+-
  err : Scope  NumInputPorts=2
  ud : Outport
  uq : Outport  Port=2
  wires:
  iq_fdb/1 -> Sum1/2
  Sum1/1 -> PID Controller1/1, err/2  "iq_err"
  id_fdb/1 -> Scope/2, Sum/2
  Sum/1 -> err/1, PID Controller/1  "id_err"
  id_ref/1 -> Scope/1, Sum/1
  iq_ref/1 -> Sum1/1
  PID Controller1/1 -> Scope1/2, uq/1  "uq"
  PID Controller/1 -> Scope1/1, ud/1  "ud"

== system OEW_PMSM_DI_SVPWM_ZSC_Control/DI_SVPWM/Sector_Calculate ==
  ualpha : Inport
  ubeta : Inport  Port=2
  MATLAB Function : MATLAB Function  TreatAsAtomicUnit=on
  N : Outport
  sector : Outport  Port=2
  wires:
  ualpha/1 -> MATLAB Function/1(ualpha)
  ubeta/1 -> MATLAB Function/2(ubeta)
  MATLAB Function/1(N) -> N/1
  MATLAB Function/2(sector) -> sector/1

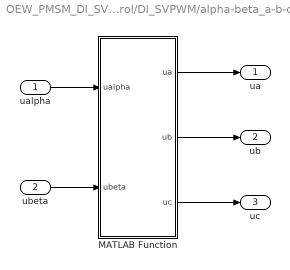
== system OEW_PMSM_DI_SVPWM_ZSC_Control/DI_SVPWM/alpha-beta_a-b-c ==
  ualpha : Inport
  ubeta : Inport  Port=2
  MATLAB Function : MATLAB Function  TreatAsAtomicUnit=on
  ua : Outport
  ub : Outport  Port=2
  uc : Outport  Port=3
  wires:
  ualpha/1 -> MATLAB Function/1(ualpha)
  ubeta/1 -> MATLAB Function/2(ubeta)
  MATLAB Function/1(ua) -> ua/1
  MATLAB Function/2(ub) -> ub/1
  MATLAB Function/3(uc) -> uc/1

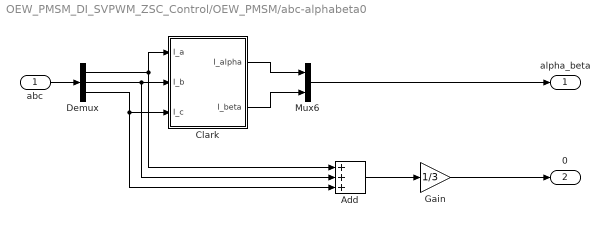
== system OEW_PMSM_DI_SVPWM_ZSC_Control/OEW_PMSM/abc-alphabeta0 ==
  abc : Inport
  Add : Sum  Inputs=+++
  Clark : Subsystem
  Demux : Demux  Outputs=3
  Gain : Gain  Gain=1/3
  Mux6 : Mux  Inputs=2
  alpha_beta : Outport  VectorParamsAs1DForOutWhenUnconnected=off
  0 : Outport  Port=2  VectorParamsAs1DForOutWhenUnconnected=off
  wires:
  Clark/2(I_beta) -> Mux6/2
  Mux6/1 -> alpha_beta/1
  Demux/3 -> Clark/3(I_c), Add/3
  Clark/1(I_alpha) -> Mux6/1
  abc/1 -> Demux/1
  Demux/2 -> Add/2, Clark/2(I_b)
  Demux/1 -> Clark/1(I_a), Add/1
  Add/1 -> Gain/1
  Gain/1 -> 0/1

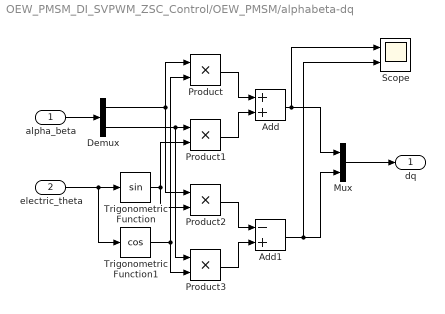
== system OEW_PMSM_DI_SVPWM_ZSC_Control/OEW_PMSM/alphabeta-dq ==
  alpha_beta : Inport
  electric_theta : Inport  Port=2
  Add : Sum
  Add1 : Sum  Inputs=-+
  Demux : Demux  Outputs=2
  Mux : Mux  Inputs=2
  Product{,1..3} (4 alike) : Product
  Scope : Scope  NumInputPorts=2
  Trigonometric Function : Trigonometry
  Trigonometric Function1 : Trigonometry  Operator=cos
  dq : Outport
  wires:
  electric_theta/1 -> Trigonometric Function1/1, Trigonometric Function/1
  Trigonometric Function1/1 -> Product3/2, Product/2
  Demux/2 -> Product3/1, Product1/1
  Trigonometric Function/1 -> Product2/2, Product1/2
  Product/1 -> Add/1
  Product1/1 -> Add/2
  Product2/1 -> Add1/1
  Product3/1 -> Add1/2
  Add/1 -> Scope/1, Mux/1
  Add1/1 -> Scope/2, Mux/2
  Demux/1 -> Product/1, Product2/1
  alpha_beta/1 -> Demux/1
  Mux/1 -> dq/1

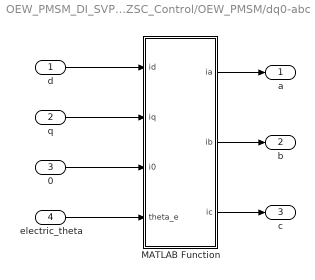
== system OEW_PMSM_DI_SVPWM_ZSC_Control/OEW_PMSM/dq0-abc ==
  d : Inport
  q : Inport  Port=2
  0 : Inport  Port=3
  electric_theta : Inport  Port=4
  MATLAB Function : MATLAB Function  TreatAsAtomicUnit=on
  a : Outport
  b : Outport  Port=2
  c : Outport  Port=3
  wires:
  d/1 -> MATLAB Function/1(id)
  q/1 -> MATLAB Function/2(iq)
  0/1 -> MATLAB Function/3(i0)
  electric_theta/1 -> MATLAB Function/4(theta_e)
  MATLAB Function/1(ia) -> a/1
  MATLAB Function/2(ib) -> b/1
  MATLAB Function/3(ic) -> c/1

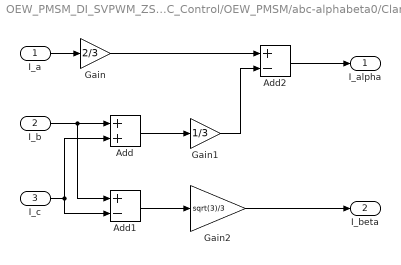
== system OEW_PMSM_DI_SVPWM_ZSC_Control/OEW_PMSM/abc-alphabeta0/Clark ==
  I_a : Inport
  I_b : Inport  Port=2
  I_c : Inport  Port=3
  Add : Sum
  Add1 : Sum  Inputs=+-
  Add2 : Sum  Inputs=+-
  Gain : Gain  Gain=2/3
  Gain1 : Gain  Gain=1/3
  Gain2 : Gain  Gain=sqrt(3)/3
  I_alpha : Outport
  I_beta : Outport  Port=2
  wires:
  I_a/1 -> Gain/1
  I_b/1 -> Add1/1, Add/1
  I_c/1 -> Add/2, Add1/2
  Add/1 -> Gain1/1
  Add1/1 -> Gain2/1
  Gain/1 -> Add2/1
  Gain1/1 -> Add2/2
  Add2/1 -> I_alpha/1
  Gain2/1 -> I_beta/1

== matlab function OEW_PMSM_DI_SVPWM_ZSC_Control/DI_SVPWM/D_Caculate ==
  data: Ma input; Ma1 output; Mb input; Mc input; sector input; tpwm input; Mb1 output; Mc1 output; Ma2 output; Mb2 output; Mc2 output
function [Ma1,Mb1,Mc1,Ma2,Mb2,Mc2] = fcn(Ma,Mb,Mc,sector,tpwm)

if sector == 1
    Ma1 = tpwm;
    Mb1 = 0;
    Mc1 = 0;
    Ma2 = Ma1 - Ma;
    Mb2 = Mb1 - Mb;
    Mc2 = Mc1 - Mc;
elseif sector == 3
    Ma1 = 0;
    Mb1 = tpwm;
    Mc1 = 0;
    Ma2 = Ma1 - Ma;
    Mb2 = Mb1 - Mb;
    Mc2 = Mc1 - Mc;
elseif sector == 5
    Ma1 = 0;
    Mb1 = 0;
    Mc1 = tpwm;
    Ma2 = Ma1 - Ma;
    Mb2 = Mb1 - Mb;
    Mc2 = Mc1 - Mc;
elseif sector == 2
    Ma2 = 0;
    Mb2 = 0;
    Mc2 = tpwm;
    Ma1 = Ma2 + Ma;
    Mb1 = Mb2 + Mb;
    Mc1 = Mc2 + Mc;
elseif sector == 4
    Ma2 = tpwm;
    Mb2 = 0;
    Mc2 = 0;
    Ma1 = Ma2 + Ma;
    Mb1 = Mb2 + Mb;
    Mc1 = Mc2 + Mc;
elseif sector == 6
    Ma2 = 0;
    Mb2 = tpwm;
    Mc2 = 0;
    Ma1 = Ma2 + Ma;
    Mb1 = Mb2 + Mb;
    Mc1 = Mc2 + Mc;
else 
    Ma1 = tpwm;
    Mb1 = 0;
    Mc1 = 0;
    Ma2 = Ma1 - Ma;
    Mb2 = Mb1 - Mb;
    Mc2 = Mc1 - Mc;
end

== matlab function OEW_PMSM_DI_SVPWM_ZSC_Control/OEW_PMSM/dq0-abc/MATLAB Function ==
  data: id input; ia output; iq input; i0 input; theta_e input; ib output; ic output
function [ia,ib,ic] = fcn(id,iq,i0,theta_e)

ia = id * cos(theta_e) - iq * sin(theta_e) + i0;
ib = id * cos(theta_e - 2*pi/3) - iq * sin(theta_e - 2*pi/3) + i0;
ic = id * cos(theta_e + 2*pi/3) - iq * sin(theta_e + 2*pi/3) + i0;

== matlab function OEW_PMSM_DI_SVPWM_ZSC_Control/DI_SVPWM/Mabc_Caculate ==
  data: ua input; Ma output; ub input; uc input; u0 input; tpwm input; udc input; Mb output; Mc output
function [Ma,Mb,Mc] = fcn(ua,ub,uc,u0,tpwm,udc)

M0 = u0 * tpwm / udc;
Ma = (ua * tpwm / udc) + M0;
Mb = (ub * tpwm / udc) + M0;
Mc = (uc * tpwm / udc) + M0;

== matlab function OEW_PMSM_DI_SVPWM_ZSC_Control/DI_SVPWM/Sector_Calculate/MATLAB Function ==
  data: ualpha input; N output; ubeta input; sector output
function [N, sector] = fcn(ualpha,ubeta)

ug = (sqrt(3)/2) * ualpha - 0.5 * ubeta;
uh = 0.5 * ualpha + (sqrt(3)/2) * ubeta;

u_ref1 = uh;
u_ref2 = -0.5 * uh + (sqrt(3)/2) * ug;
u_ref3 = -0.5 * uh - (sqrt(3)/2) * ug;

if u_ref1 > 0
    A = 1;
else
    A = 0;
end

if u_ref2 > 0
    B = 1;
else
    B = 0;
end

if u_ref3 > 0
    C = 1;
else
    C = 0;
end

n = A + 2 * B + 4 * C;

if n == 0
    N = 1;
else
    N = n;
end

if N == 1
    sector = 2;
elseif N == 2
    sector = 6;
elseif N == 3
    sector = 1;
elseif N == 4
    sector = 4;
elseif N == 5
    sector = 3;
elseif N == 6
    sector = 5;
else 
    sector = 2;
end

== matlab function OEW_PMSM_DI_SVPWM_ZSC_Control/ZSC_Controller/MATLAB Function ==
  data: ref input; output output; fdb input; we input; Ts input
function output = fcn(ref, fdb, we, Ts)

Kp = 20.0;      % 比例增益
Ki = 1000.0;    % 谐振增益

% 计算误差
e = ref - fdb;

% 比例部分
output_p = Kp * e;

% 谐振部分
% 使用双线性变换进行离散化

% 谐振频率
wr = 3 * we;

% 避免除零错误
if abs(wr) < 1e-6
    output_r = 0;
    output = output_p;
    return;
end

% 计算中间变量
T = Ts;
a = wr^2;
b = 4/T^2 + a;
b0 = (2*Ki/T) / b;
b1 = 0;
b2 = -b0;
a1 = (2*a - 8/T^2) / b;
a2 = (4/T^2 - 2*a + wr^2*T^2) / b;

% 使用持久变量存储历史状态
persistent x_r_prev1 x_r_prev2 e_r_prev1 e_r_prev2;
if isempty(x_r_prev1)
    x_r_prev1 = 0;
    x_r_prev2 = 0;
    e_r_prev1 = 0;
    e_r_prev2 = 0;
end

% 谐振部分差分方程
output_r = b0*e + b1*e_r_prev1 + b2*e_r_prev2 - a1*x_r_prev1 - a2*x_r_prev2;

% 更新状态变量
e_r_prev2 = e_r_prev1;
e_r_prev1 = e;
x_r_prev2 = x_r_prev1;
x_r_prev1 = output_r;

output = output_p + output_r;

end

== matlab function OEW_PMSM_DI_SVPWM_ZSC_Control/DI_SVPWM/alpha-beta_a-b-c/MATLAB Function ==
  data: ualpha input; ua output; ubeta input; ub output; uc output
function [ua,ub,uc] = fcn(ualpha,ubeta)

ua = ualpha;
ub = -0.5 * ualpha + (sqrt(3)/2) * ubeta;
uc = -0.5 * ualpha - (sqrt(3)/2) * ubeta;
